simulink model "buckboost"  (R2022b)
settings: Solver=VariableStepAuto  StartTime=0.0  StopTime=1  RelTol=1e-3
libraries: spsCurrentMeasurementLib x6, spsVoltageMeasurementLib x4, spsParallelRLCBranchLib x3, spsDCVoltageSourceLib x1, spsDiodeLib x1, spsMeanLib x1, spsMosfetLib x1, sps_lib x1
settings Model: Creator=isild  LastModifiedBy=isild

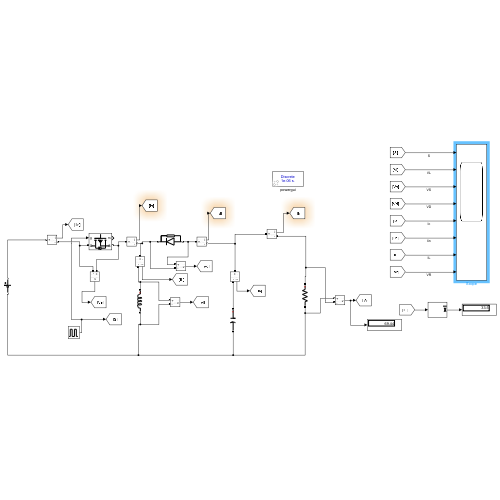
[thumbnail: Simulink's stored preview of the top-level diagram]
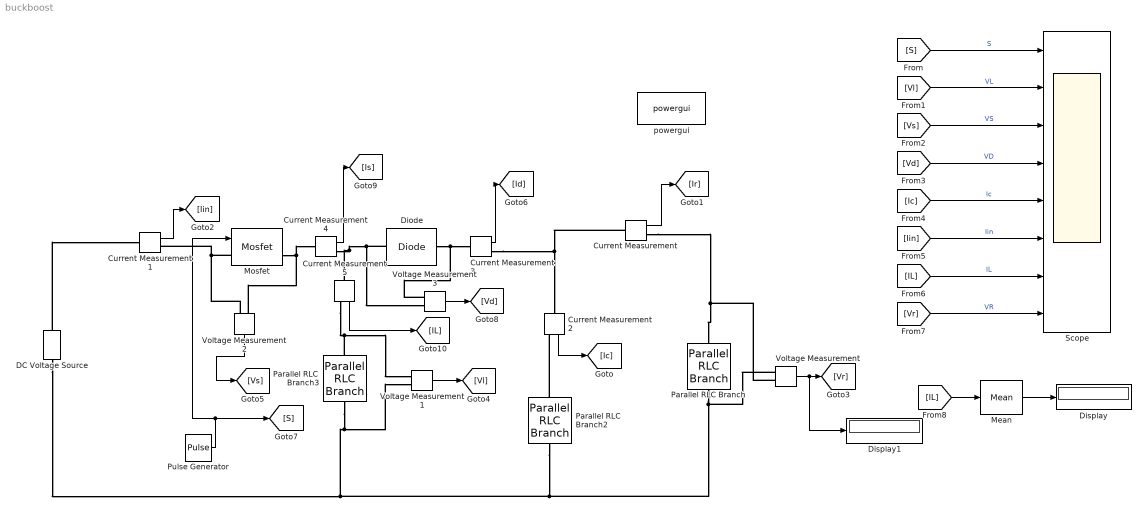
== system buckboost ==
  Current Measurement{,1..5} (6 alike) : spsCurrentMeasurementLib/Current Measurement  PhasorSimulation=off  OutputType=Complex  PSBequivalent=0
  DC Voltage Source : spsDCVoltageSourceLib/DC Voltage Source  Amplitude=50  Measurements=None
  Diode : spsDiodeLib/Diode  Ron=0.001  Lon=0  Vf=0.8  IC=0  UseSnubber=0  Rs=500  Cs=250e-9  Measurements=off
  Display : Display
  Display1 : Display
  Mean : spsMeanLib/Mean  Freq=60  Vinit=0  Ts=0
  Mosfet : spsMosfetLib/Mosfet  Ron=0.1  Lon=0  Rd=0.01  Vfd=0  IC=0  Rs=1e5  Cs=inf  Measurements=on
  Parallel RLC Branch : spsParallelRLCBranchLib/Parallel RLC Branch  LConnTagsString=a  RConnTagsString=__new0  BranchType=R  Resistance=5.18  Inductance=1e-3  SetiL0=off  InitialCurrent=0  Capacitance=1e-6  Setx0=off  InitialVoltage=0  Measurements=None
  Parallel RLC Branch2 : spsParallelRLCBranchLib/Parallel RLC Branch  LConnTagsString=a  RConnTagsString=__new0  BranchType=C  Resistance=1  Inductance=1e-3  SetiL0=off  InitialCurrent=0  Capacitance=569e-6  Setx0=off  InitialVoltage=0  Measurements=None
  Parallel RLC Branch3 : spsParallelRLCBranchLib/Parallel RLC Branch  LConnTagsString=a  RConnTagsString=__new0  BranchType=L  Resistance=1  Inductance=145e-6  SetiL0=off  InitialCurrent=0  Capacitance=1e-6  Setx0=off  InitialVoltage=0  Measurements=None
  Pulse Generator : DiscretePulseGenerator  PulseType=Time based  Period=1/20000  PulseWidth=59
  Scope : Scope  NumInputPorts=8
  Voltage Measurement{,1..3} (4 alike) : spsVoltageMeasurementLib/Voltage Measurement  PhasorSimulation=off  OutputType=Complex  PSBequivalent=0
  powergui : sps_lib/powergui  Priority=1  SimulationMode=Discrete  SampleTime=1e-6  frequency=60  Iterations=50  frequencyindice=0  Pbase=100e6  ErrMax=1e-4  UnitsV=kV  UnitsW=MW  buscounter=0  FunctionMessages=off  echomessages=off  EnableUseOfTLC=off  CurrentSourceSwitches=off  DisableSnubberDevices=off  DisableRonSwitches=off  DisableVfSwitches=off  DisplayEquations=off  AutomaticDiscreteSolvers=off  SolverType=Tustin/Backward Euler (TBE)  Interpol=off  ExternalGateDelay=off  methode=off  Ts=100  x0status=blocks  SPID=on  SwTol=0  HookPort=off  NonlinearTolerance=1e-4  nMaxIteration=100  ContinueOnMaxIteration=off  RestoreLinks=warning  ResistiveCurrentMeasurement=off  Frange=[0:2:500]  Ylog=off  Xlog=on  ShowGrid=off  save=off  variable=ZData  structure=0  ZoomFFT=off  StartTime=0.0  cycles=1  DisplayStyle=1  fundamental=60  FreqAxis=off  MaxFrequency=1000  frequencyindicesteady=1  RmsSteady=1  display=off
  wires:
  Current Measurement4/1 -> [Is]
  Voltage Measurement1/1 -> [Vl]
  Current Measurement3/1 -> [Id]
  Current Measurement2/1 -> [Ic]
  Current Measurement/1 -> [Ir]
  Voltage Measurement/1 -> Display1/1, [Vr]
  Voltage Measurement2/1 -> [Vs]
  Pulse Generator/1 -> [S], Mosfet/1
  Current Measurement1/1 -> [Iin]
  Voltage Measurement3/1 -> [Vd]
  [S] -> Scope/1  "S"
  [Vl] -> Scope/2  "VL"
  [Vs] -> Scope/3  "VS"
  [Vd] -> Scope/4  "VD"
  [Ic] -> Scope/5  "Ic"
  [Iin] -> Scope/6  "Iin"
  [IL] -> Scope/7  "IL"
  [Vr] -> Scope/8  "VR"
  Current Measurement5/1 -> [IL]
  [IL] -> Mean/1
  Mean/1 -> Display/1
  connections:
  Current Measurement3/RConn1 -- Current Measurement2/LConn1 -- Current Measurement/LConn1
  Parallel RLC Branch/RConn1 -- Parallel RLC Branch2/RConn1 -- DC Voltage Source/LConn1 -- Parallel RLC Branch3/RConn1 -- Voltage Measurement1/LConn2 -- Voltage Measurement/LConn1
  Voltage Measurement3/LConn1 -- Diode/LConn1 -- Current Measurement3/LConn1
  Voltage Measurement2/LConn2 -- Current Measurement1/RConn1 -- Mosfet/LConn1
  Current Measurement4/RConn1 -- Current Measurement5/LConn1 -- Diode/RConn1 -- Voltage Measurement3/LConn2
  Voltage Measurement2/LConn1 -- Current Measurement4/LConn1 -- Mosfet/RConn1
  Current Measurement/RConn1 -- Voltage Measurement/LConn2 -- Parallel RLC Branch/LConn1
  DC Voltage Source/RConn1 -- Current Measurement1/LConn1
  Parallel RLC Branch2/LConn1 -- Current Measurement2/RConn1
  Parallel RLC Branch3/LConn1 -- Voltage Measurement1/LConn1 -- Current Measurement5/RConn1
